simulink model "pos_cont"  (R2014a)
settings: Solver=FixedStepDiscrete  StartTime=0.0  StopTime=inf  FixedStep=sample_time  RelTol=1e-3
values from neighbouring files (symbols this model uses):
  hip_d = 5    [pos_cont_params.m]
  hip_p = 50    [pos_cont_params.m]
  hip_sat = 50    [pos_cont_params.m]
  leg_d = 5    [pos_cont_params.m]
  leg_p = 50    [pos_cont_params.m]
  leg_sat = 50    [pos_cont_params.m]
settings Model: xpc_rtwmakecfg_data=_xpcethercatlib_  BufferReuse=off  Creator=wmartin  LastModifiedBy=ryan
settings SolverCC: EnableConcurrentExecution=on
settings DataIOCC: MaxDataPoints=1000000000  SaveFormat=StructureWithTime  SaveOutput=off  SaveTime=off
settings OptimizationCC: BlockReduction=off  OptimizeBlockIOStorage=off  BufferReuse=off  GlobalBufferReuse=off  ExpressionFolding=off  ExpressionDepthLimit=2147483647  LocalBlockOutputs=off  SimCompilerOptimization=On
settings DebuggingCC: UnderspecifiedInitializationDetection=Classic  StateNameClashWarn=warning
settings HardwareCC: ProdIntDivRoundTo=Zero  ProdEndianess=LittleEndian  ProdHWDeviceType=Generic->32-bit x86 compatible
settings ModelReferenceCC: UpdateModelReferenceTargets=IfOutOfDate  ModelReferenceNumInstancesAllowed=Single  ModelReferenceMinAlgLoopOccurrences=on
settings RTWCC: SystemTargetFile=slrt.tlc  TemplateMakefile=slrt_default_tmf  Description=Simulink Real-Time  RTWVerbose=off  ProcessScript=slrt_make_rtw_hook  RTWCompilerOptimization=On
settings SimulinkRealTimeCC: GeneratePreprocessorConditionals=Disable all  EnableShiftOperators=on  RL32LogBufSizeModifier=100000000

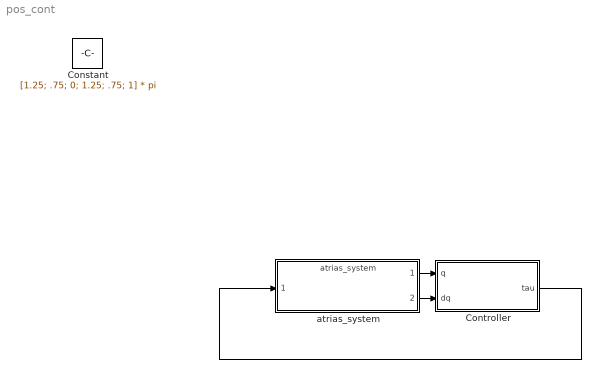
== system pos_cont ==
  Controller : Subsystem
  atrias_system : ModelReference  ModelNameDialog=atrias_system  SimulationMode=Normal  ModelReferenceVersion=1.1560  CopyOfModelName=atrias_system  DefaultDataLogging=on
  Constant : Constant  IOType=siggen  Value=[1.25; .75; 0; 1.25; .75; 1] * pi
  wires:
  atrias_system/1 -> Controller/1(q)
  atrias_system/2 -> Controller/2(dq)
  Controller/1(tau) -> atrias_system/1

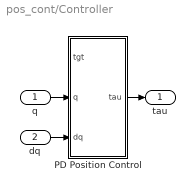
== system pos_cont/Controller ==
  q : Inport
  dq : Inport  Port=2
  PD Position Control : MATLAB Function  TreatAsAtomicUnit=on
  tau : Outport
  wires:
  PD Position Control/1(tau) -> tau/1
  q/1 -> PD Position Control/2(q)
  dq/1 -> PD Position Control/3(dq)

== matlab function pos_cont/Controller/PD Position Control ==
  data: tgt input; tau output; q input; dq input; hip_sat parameter; leg_sat parameter; leg_p parameter; leg_d parameter; hip_p parameter; hip_d parameter
function tau = fcn(tgt, q, dq, hip_sat, leg_sat, leg_p, leg_d, hip_p, hip_d)
%#codegen

% Grab motor positions and velocities
motors = [2 4 9 6 8 10];
mot_q  = q( motors);
mot_dq = dq(motors);

% Initialize the output
tau = zeros(6,1);

% Do the control
tau = [leg_p; leg_p; hip_p; leg_p; leg_p; hip_p] .* (tgt - mot_q) - ...
      [leg_d; leg_d; hip_d; leg_d; leg_d; hip_d] .* mot_dq;

% Apply the saturation limits
all_sats = [leg_sat; leg_sat; hip_sat; leg_sat; leg_sat; hip_sat];
tau      = min(tau,  all_sats);
tau      = max(tau, -all_sats);
